simulink model "Ball_Detection_and_PID"  (R2020a)
settings: Solver=ode3  StartTime=0.0  StopTime=inf  FixedStep=1/30  RelTol=1e-3
values from neighbouring files (symbols this model uses):
  AValues = griddata(data.alpha,data.beta,data.AngleservoA,Alpha,Beta)    [dataToLookupTable.m]
  BValues = griddata(data.alpha,data.beta,data.AngleservoB,Alpha,Beta)    [dataToLookupTable.m]
  CValues = griddata(data.alpha,data.beta,data.AngleservoC,Alpha,Beta)    [dataToLookupTable.m]
undefined symbols (not defined in the file or in its folder): none, serial, videoinput
libraries: simulink x2, instrumentlib x2, svdutilitieslib x1, visiontextngfix x1, imaqlib x1, visionsinks x1
settings Model: Creator=vince  LastModifiedBy=vince

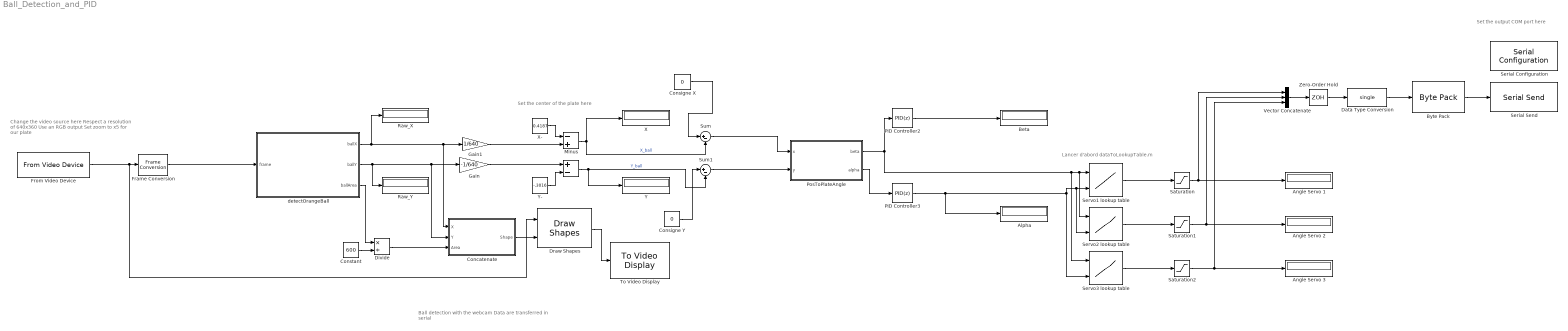
== system Ball_Detection_and_PID ==
  note: Set the center of the plate here
  note: Set the output COM port here
  note: Change the video source here
      | Respect a resolution of 640x360
      | Use an RGB output
      | Set zoom to x5 for our plate
  note: Ball detection with the webcam
      | Data are transferred in serial
  note: Lancer d'abord dataToLookupTable.m
  " " : Sum  Inputs=+-
  Alpha : Display
  Angle Servo 1 : Display
  Angle Servo 2 : Display
  Angle Servo 3 : Display
  Beta : Display
  Byte Pack : svdutilitieslib/Byte Pack  maskPackedDataType=uint32  datatypes={'single'}  byteAlign=4  blockPlatform=arduinoert
      settings: SourceProductBaseCode=ARDUINO,ML_ARDUINO,ECCORTEXA,ECCORTEXR,SC_BEAGLEBONE_BLUE,EC_FREEDOM_BOARD,EC_FRDM_K64F,INTEL_BLOCKSET,MICROBIT,NUCLEO,PX4AUTOPILOTS,RASPPIIO,STMICRODIS,TIC2000,XILINX_BLOCKSET
  Concatenate : MATLAB Function  TreatAsAtomicUnit=on
  Consigne X : Constant  Value=0
  Consigne Y : Constant  Value=0
  Constant : Constant  Value=600
  Data Type Conversion : DataTypeConversion  OutDataTypeStr=single
  Divide : Product  Inputs=*/
  Draw Shapes : visiontextngfix/Draw Shapes  shape=Circles  fill=on  lineWidth=1  fillClrSource=Specify via dialog  display=User-specified value  intensity=200  color=[255 255 000]  opacity=0.6  viewport=Entire image  antialiasing=off  inType=Obsolete  imagePorts=One multidimensional signal  roundingMode=Floor  overflowMode=off  memoryMode=Specify word length  memoryWordLength=16  prodOutputMode=Binary point scaling  prodOutputWordLength=32  prodOutputFracLength=14  memoryFracLength=15
  Frame Conversion : FrameConversion  OutFrame=Sample-based
  From Video Device : imaqlib/From Video Device  DeviceMenu=winvideo 1 (Microsoft® LifeCam HD-3000)  Device=winvideo 1 (Microsoft® LifeCam HD-3000)  ObjConstructor=videoinput('winvideo', 1)  VideoFormatMenu=YUY2_640x360  VideoFormat=YUY2_640x360  VideoSource=input1  ROIPosition=[0 0 360 640]  EnableHWTrigger=off  TriggerConfiguration=none/none  SampleTime=1/30  OutputPortsMode=One multidimensional signal  DataType=single  CanDoHWTrigger=no  ReturnedColorSpace=rgb  BlockHandle=32.0001  ROIWidth=640  ROIHeight=360  ROIColumn=0  ROIRow=0  EngXMLPath=C:\Program Files\MATLAB\R2020a\toolbox\imaq\imaq\private  DevXMLPath=C:\ProgramData\MATLAB\SupportPackages\R2020a\toolbox\imaq\supportpackages\genericvideo\adaptor\win64  EngLibPath=C:\Program Files\MATLAB\R2020a\toolbox\imaq\imaqblks\imaqmex\win64  ColorSpace=rgb  BayerSensorAlignment=grbg  ImaqMode=off
  Gain : Gain  Gain=-1/640
  Gain1 : Gain  Gain=1/640
  Minus : Sum  Inputs=-+
  PID Controller2 : simulink/Continuous/PID Controller  Controller=PID  Form=Parallel  TimeDomain=Discrete-time  UseExternalTs=off  SampleTime=-1  IntegratorMethod=Forward Euler  FilterMethod=Forward Euler  ControllerParametersSource=internal  P=2  I=0  D=0  UseFilter=off  N=100  TunerSelectOption=Transfer Function Based (PID Tuner App)  InitialConditionSource=internal  InitialConditionForIntegrator=0  InitialConditionForFilter=0  DifferentiatorICPrevScaledInput=0  ExternalReset=none  TrackingMode=off  Kt=1  LimitOutput=off  UpperSaturationLimit=inf  LowerSaturationLimit=-inf  LinearizeAsGain=on  AntiWindupMode=none  Kb=1  POutMin=[]  POutMax=[]  IOutMin=[]  IOutMax=[]  DOutMin=[]  DOutMax=[]  NOutMin=[]  NOutMax=[]  SumOutMin=[]  SumOutMax=[]  SaturationOutMin=[]  SaturationOutMax=[]  PParamMin=[]  PParamMax=[]  IParamMin=[]  IParamMax=[]  DParamMin=[]  DParamMax=[]  NParamMin=[]  NParamMax=[]  KbParamMin=[]  KbParamMax=[]  KtParamMin=[]  KtParamMax=[]  KbOutMin=[]  KbOutMax=[]  KtOutMin=[]  KtOutMax=[]  IntegratorOutMin=[]  IntegratorOutMax=[]  FilterOutMin=[]  FilterOutMax=[]  SumI1OutMin=[]  SumI1OutMax=[]  SumI2OutMin=[]  SumI2OutMax=[]  SumI3OutMin=[]  SumI3OutMax=[]  SumI4OutMin=[]  SumI4OutMax=[]  SumDOutMin=[]  SumDOutMax=[]  DifferentiatorOutMin=[]  DifferentiatorOutMax=[]  FilterDiffOutCoefMin=[]  FilterDiffOutCoefMax=[]  ReciprocalOutMin=[]  ReciprocalOutMax=[]  SumDenOutMin=[]  SumDenOutMax=[]  SumNumOutMin=[]  SumNumOutMax=[]  DivideOutMin=[]  DivideOutMax=[]  UdiffTsProdOutMin=[]  UdiffTsProdOutMax=[]  NTsProdOutMin=[]  NTsProdOutMax=[]  UintegralTsProdOutMin=[]  UintegralTsProdOutMax=[]  UngainTsProdOutMin=[]  UngainTsProdOutMax=[]  IntegratorContinuousStateAttributes=''  IntegratorStateMustResolveToSignalObject=off  IntegratorRTWStateStorageClass=Auto  FilterContinuousStateAttributes=''  FilterStateMustResolveToSignalObject=off  FilterRTWStateStorageClass=Auto  ParallelPVariant=InternalParameters  IdealPVariant=Disabled  IVariant=InternalParameters  DVariant=InternalParameters  IntegratorVariant=Discrete  SatVariant=Disabled  AWVariant=Passthrough  PCopyVariant=Disabled  TRVariant=Disabled  FdbkBlocksVariant=Forward  IdealPFdbkVariant=Disabled  SatFdbkVariant=Disabled  DerivativeFilterVariant=Differentiator  NVariant=Passthrough  NCopyVariant=Disabled_SignalSpec  FilterICVariant=InternalICsDifferentiator  IntegratorICVariant=InternalICs  ExternalResetVariant=Disabled  TRSumVariant=Passthrough  SumFdbkVariant=Disabled  SumVariant=Sum_PID  TsampFilterVariant=InternalTs  TsampNgainVariant=Passthrough  TsampIntegralVariant=Passthrough
  PID Controller3 : simulink/Continuous/PID Controller  Controller=PID  Form=Parallel  TimeDomain=Discrete-time  UseExternalTs=off  SampleTime=-1  IntegratorMethod=Forward Euler  FilterMethod=Forward Euler  ControllerParametersSource=internal  P=2  I=0  D=0  UseFilter=off  N=100  TunerSelectOption=Transfer Function Based (PID Tuner App)  InitialConditionSource=internal  InitialConditionForIntegrator=0  InitialConditionForFilter=0  DifferentiatorICPrevScaledInput=0  ExternalReset=none  TrackingMode=off  Kt=1  LimitOutput=off  UpperSaturationLimit=inf  LowerSaturationLimit=-inf  LinearizeAsGain=on  AntiWindupMode=none  Kb=1  POutMin=[]  POutMax=[]  IOutMin=[]  IOutMax=[]  DOutMin=[]  DOutMax=[]  NOutMin=[]  NOutMax=[]  SumOutMin=[]  SumOutMax=[]  SaturationOutMin=[]  SaturationOutMax=[]  PParamMin=[]  PParamMax=[]  IParamMin=[]  IParamMax=[]  DParamMin=[]  DParamMax=[]  NParamMin=[]  NParamMax=[]  KbParamMin=[]  KbParamMax=[]  KtParamMin=[]  KtParamMax=[]  KbOutMin=[]  KbOutMax=[]  KtOutMin=[]  KtOutMax=[]  IntegratorOutMin=[]  IntegratorOutMax=[]  FilterOutMin=[]  FilterOutMax=[]  SumI1OutMin=[]  SumI1OutMax=[]  SumI2OutMin=[]  SumI2OutMax=[]  SumI3OutMin=[]  SumI3OutMax=[]  SumI4OutMin=[]  SumI4OutMax=[]  SumDOutMin=[]  SumDOutMax=[]  DifferentiatorOutMin=[]  DifferentiatorOutMax=[]  FilterDiffOutCoefMin=[]  FilterDiffOutCoefMax=[]  ReciprocalOutMin=[]  ReciprocalOutMax=[]  SumDenOutMin=[]  SumDenOutMax=[]  SumNumOutMin=[]  SumNumOutMax=[]  DivideOutMin=[]  DivideOutMax=[]  UdiffTsProdOutMin=[]  UdiffTsProdOutMax=[]  NTsProdOutMin=[]  NTsProdOutMax=[]  UintegralTsProdOutMin=[]  UintegralTsProdOutMax=[]  UngainTsProdOutMin=[]  UngainTsProdOutMax=[]  IntegratorContinuousStateAttributes=''  IntegratorStateMustResolveToSignalObject=off  IntegratorRTWStateStorageClass=Auto  FilterContinuousStateAttributes=''  FilterStateMustResolveToSignalObject=off  FilterRTWStateStorageClass=Auto  ParallelPVariant=InternalParameters  IdealPVariant=Disabled  IVariant=InternalParameters  DVariant=InternalParameters  IntegratorVariant=Discrete  SatVariant=Disabled  AWVariant=Passthrough  PCopyVariant=Disabled  TRVariant=Disabled  FdbkBlocksVariant=Forward  IdealPFdbkVariant=Disabled  SatFdbkVariant=Disabled  DerivativeFilterVariant=Differentiator  NVariant=Passthrough  NCopyVariant=Disabled_SignalSpec  FilterICVariant=InternalICsDifferentiator  IntegratorICVariant=InternalICs  ExternalResetVariant=Disabled  TRSumVariant=Passthrough  SumFdbkVariant=Disabled  SumVariant=Sum_PID  TsampFilterVariant=InternalTs  TsampNgainVariant=Passthrough  TsampIntegralVariant=Passthrough
  PosToPlateAngle : MATLAB Function  TreatAsAtomicUnit=on
  Raw_X : Display
  Raw_Y : Display
  Saturation : Saturate  UpperLimit=50  LowerLimit=0
  Saturation1 : Saturate  UpperLimit=50  LowerLimit=0
  Saturation2 : Saturate  UpperLimit=50  LowerLimit=0
  Serial Configuration : instrumentlib/Serial Configuration  Priority=-200000  ComPortMenu=COM6  ComPort=COM6  ObjConstructor=serial('COM6');  BaudRate=115200  DataBits=8  Parity=none  StopBits=1  FlowControl=none  Timeout=10  ByteOrder=LittleEndian
  Serial Send : instrumentlib/Serial Send  ComPortMenu=COM6  ComPort=COM6  ObjConstructor=serial('COM6');  Terminator=<none>  EnableBlockingMode=on
  Servo1 lookup table : Lookup_n-D  BreakpointsSpecification=Even spacing  BreakpointsForDimension1=[1:1801]  BreakpointsForDimension2=[1:176]  BreakpointsForDimension3=[2:316988]  BreakpointsForDimension1FirstPoint=0  BreakpointsForDimension2FirstPoint=0  BreakpointsForDimension1Spacing=0.2  BreakpointsForDimension2Spacing=0.2  IndexSearchMethod=Evenly spaced points  Table=AValues  TableDataTypeStr=Inherit: Inherit from 'Table data'  InterpMethod=Nearest  InternalRulePriority=Speed  OutMin=[3]  OutMax=[3]  OutDataTypeStr=double  RndMeth=Simplest  InputSameDT=on
  Servo2 lookup table : Lookup_n-D  BreakpointsSpecification=Even spacing  BreakpointsForDimension1=[1:1801]  BreakpointsForDimension2=[1:176]  BreakpointsForDimension3=[2:316988]  BreakpointsForDimension1FirstPoint=0  BreakpointsForDimension2FirstPoint=0  BreakpointsForDimension1Spacing=0.2  BreakpointsForDimension2Spacing=0.2  IndexSearchMethod=Evenly spaced points  Table=BValues  TableDataTypeStr=Inherit: Inherit from 'Table data'  InterpMethod=Nearest  InternalRulePriority=Speed  OutMin=[3]  OutMax=[3]  OutDataTypeStr=double  RndMeth=Simplest  InputSameDT=on
  Servo3 lookup table : Lookup_n-D  BreakpointsSpecification=Even spacing  BreakpointsForDimension1=[1:1801]  BreakpointsForDimension2=[1:176]  BreakpointsForDimension3=[2:316988]  BreakpointsForDimension1FirstPoint=0  BreakpointsForDimension2FirstPoint=0  BreakpointsForDimension1Spacing=0.2  BreakpointsForDimension2Spacing=0.2  IndexSearchMethod=Evenly spaced points  Table=CValues  TableDataTypeStr=Inherit: Inherit from 'Table data'  InterpMethod=Nearest  InternalRulePriority=Speed  OutMin=[3]  OutMax=[3]  OutDataTypeStr=double  RndMeth=Simplest  InputSameDT=on
  Sum : Sum  Inputs=|+-
  Sum1 : Sum  Inputs=|+-
  To Video Display : visionsinks/To Video Display  windowSizeMode=Normal  openAtMdlStart=on  fullScreen=off  videoWindowX=961  videoWindowY=31  saveWindowSize=off  videoWindowWidth=958  videoWindowHeight=1008  inputColorFormat=RGB  inputType=Obsolete  imagePorts=One multidimensional signal  OutputDevice=On-screen video monitor  dataOrg=Column-major  isWindowOpen=off
  Vector Concatenate : Concatenate  NumInputs=3
  X : Display
  X- : Constant  Value=0.4187
  Y : Display
  Y- : Constant  Value=-.3016
  Zero-Order Hold : ZeroOrderHold  SampleTime=0.2
  detectOrangeBall : MATLAB Function  TreatAsAtomicUnit=on  RTWFcnName=detectOrangeBall
  wires:
  Frame Conversion/1 -> detectOrangeBall/1(frame)
  From Video Device/1 -> Draw Shapes/1, Frame Conversion/1
  detectOrangeBall/1(ballX) -> Gain1/1, Concatenate/1(X), Raw_X/1
  detectOrangeBall/3(ballArea) -> Divide/1
  Draw Shapes/1 -> To Video Display/1
  detectOrangeBall/2(ballY) -> Gain/1, Concatenate/2(Y), Raw_Y/1
  Concatenate/1(Shape) -> Draw Shapes/2
  Constant/1 -> Divide/2
  Divide/1 -> Concatenate/3(Area)
  X-/1 -> Minus/1
  Y-/1 -> " "/2
  Minus/1 -> X/1, Sum/2  "X_ball"
  " "/1 -> Sum1/2, Y/1  "Y_ball"
  Servo3 lookup table/1 -> Saturation2/1
  Servo1 lookup table/1 -> Saturation/1
  Servo2 lookup table/1 -> Saturation1/1
  Consigne X/1 -> Sum/1
  Consigne Y/1 -> Sum1/1
  Gain/1 -> " "/1
  PosToPlateAngle/1(beta) -> Servo3 lookup table/1, Servo2 lookup table/1, Servo1 lookup table/1, PID Controller2/1
  PosToPlateAngle/2(alpha) -> PID Controller3/1
  Vector Concatenate/1 -> Zero-Order Hold/1
  Sum/1 -> PosToPlateAngle/1(x)
  Sum1/1 -> PosToPlateAngle/2(y)
  Gain1/1 -> Minus/2
  PID Controller2/1 -> Beta/1
  PID Controller3/1 -> Servo3 lookup table/2, Servo2 lookup table/2, Servo1 lookup table/2, Alpha/1
  Saturation/1 -> Vector Concatenate/1, Angle Servo 1/1
  Saturation1/1 -> Vector Concatenate/2, Angle Servo 2/1
  Saturation2/1 -> Vector Concatenate/3, Angle Servo 3/1
  Zero-Order Hold/1 -> Data Type Conversion/1
  Data Type Conversion/1 -> Byte Pack/1
  Byte Pack/1 -> Serial Send/1

== matlab function Ball_Detection_and_PID/Concatenate ==
  data: X input size=1; Shape output size=[1 3]; Y input size=1; Area input size=[2]
function Shape = Concatenate(X,Y ,Area)
Shape=[int32(X(1)), int32(Y(1)), int32(Area(1))];

== matlab function Ball_Detection_and_PID/detectOrangeBall ==
  data: ballX output size=1; ballY output size=1; frame input; ballArea output size=[2]
function [ballX, ballY, ballArea] = detectOrangeBall(frame)
% Create the default minimum and maximum HSV values for orange color
orangeMin =  [0.05 0.4 0.5];
orangeMax =  [0.15 1.0 1.0];
ballArea = int32(0); % Fixed size for Simulink
DefaultX= int32(297.4);
DefaultY= int32(198.5);
% Create a blob analysis object
blobAnalyzer = vision.BlobAnalysis('MinimumBlobArea', 100, 'MaximumBlobArea', 10000);
ballX = int32(zeros(1));
ballY = int32(zeros(1));
while true
    % Check if the input frame is empty
    if isempty(frame)
        ballX = DefaultX;
        ballY = DefaultY;
        ballArea = int32(0);
        break;
    end
    
    % Convert the frame to HSV color space
    hsv = rgb2hsv(frame);
    
    % Create a mask for the orange color
    mask = (hsv(:,:,1) >= orangeMin(1)) & (hsv(:,:,1) <= orangeMax(1)) & ...
           (hsv(:,:,2) >= orangeMin(2)) & (hsv(:,:,2) <= orangeMax(2)) & ...
           (hsv(:,:,3) >= orangeMin(3)) & (hsv(:,:,3) <= orangeMax(3));
       
    % Perform blob analysis on the mask
    [areas, centroids] = step(blobAnalyzer, mask);
    
    % Find the largest blob in the image
    index = [];
    if ~isempty(areas)
        [~, index] = max(areas);
        tempX= int32(centroids(index, 1));
        ballX = tempX(1);
        tempY = int32(centroids(index, 2));
        ballY = tempY(1);
        ballArea = areas(index);
    else
        ballX = DefaultX;
        ballY = DefaultY;
        ballArea = int32(0);
        break; % No ball has been found
    end
    
    % Output the centroid and area of the largest blob
    if ~isempty(centroids)
        tempX = int32(centroids(index, 1));
        ballX = tempX(1);
        tempY = int32(centroids(index, 2));
        ballY = tempY(1);
        ballArea = areas(index);
        break;
    end
end

== matlab function Ball_Detection_and_PID/PosToPlateAngle ==
  data: beta output; x input size=1; alpha output; y input size=1
function [beta,alpha] = PosToPlateAngle(x,y)
toDeg=180/pi;
%alpha=asin(sqrt(x^2+y^2))*toDeg;

alpha = asin(x)*toDeg;;
% gamma = atan(y)*toDeg;

%gamma = atan(y/x)*toDeg;

% if (x>0 && y>=0)
%     beta=180-abs(gamma);
% elseif (x>0 && y<=0)
%     beta=180+abs(gamma);
% elseif(x<0 && y>=0)
%     beta=abs(gamma);
% elseif(x<0 && y<=0)
%     beta=360-abs(gamma);
% elseif(x==0 && y>= 0)
%     beta=90;
% else
%     beta=270;
% end

beta = asin(y)*toDeg;;
